simulink model "homework6"  (R2014b)
settings: Solver=ode45  StartTime=0.0  StopTime=10.0  RelTol=1e-3
values from neighbouring files (symbols this model uses):
  A = [-8.29e-2    0       -6.6e2   3.22e1 0, ... (first row only)    [hw6.m]
  B = [ 0      7.65, ... (first row only)    [hw6.m]
  C = [0     1 0 0 0, ... (first row only)    [hw6.m]
  D = [0 0, ... (first row only)    [hw6.m]
undefined symbols (not defined in the file or in its folder): sigbuilder_block
settings Model: Creator=karasinski  LastModifiedBy=karasinski

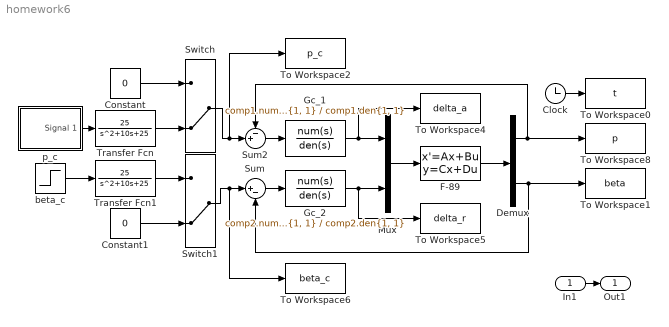
== system homework6 ==
  In1 : Inport
  Clock : Clock
  Constant : Constant  Value=0
  Constant1 : Constant  Value=0
  Demux : Demux  Outputs=2
  F-89 : StateSpace  A=A  B=B  C=C  D=D  X0=0
  Gc_1 : TransferFcn  Numerator=comp1.num{1, 1}  Denominator=comp1.den{1, 1}
  Gc_2 : TransferFcn  Numerator=comp2.num{1, 1}  Denominator=comp2.den{1, 1}
  Mux : Mux  Inputs=2
  Sum : Sum  Inputs=|+-
  Sum2 : Sum  Inputs=-+|
  Switch : ManualSwitch  CurrentSetting=0
  Switch1 : ManualSwitch  CurrentSetting=0
  To Workspace0 : ToWorkspace  VariableName=t  SampleTime=-1
  To Workspace1 : ToWorkspace  VariableName=beta  SampleTime=-1
  To Workspace2 : ToWorkspace  VariableName=p_c  SampleTime=-1
  To Workspace4 : ToWorkspace  VariableName=delta_a  SampleTime=-1
  To Workspace5 : ToWorkspace  VariableName=delta_r  SampleTime=-1
  To Workspace6 : ToWorkspace  VariableName=beta_c  SampleTime=-1
  To Workspace8 : ToWorkspace  VariableName=p  SampleTime=-1
  Transfer Fcn : TransferFcn  Numerator=[25]  Denominator=[1 10 25]
  Transfer Fcn1 : TransferFcn  Numerator=[25]  Denominator=[1 10 25]
  beta_c : Step  Time=0  After=5 / 57.3  SampleTime=0
  p_c : Subsystem  Tag=STV Subsys  LoadFcn=sigbuilder_block('load');  StartFcn=sigbuilder_block('start');  StopFcn=sigbuilder_block('stop');  ClipboardFcn=sigbuilder_block('clipboard');  mask(Sigbuilder block){}
      mask help: Simulink:masks:SigbuilderBlock_MD
      mask init:
      | if ~strcmp(get_param(bdroot(gcbh),'SimulationStatus'),'stopped') tuvar = sigbuilder_block('maskInit'); end
      settings: CopyFcn=sigbuilder_block('copy');  DeleteFcn=sigbuilder_block('delete');  ModelCloseFcn=sigbuilder_block('modelClose');  PreSaveFcn=sigbuilder_block('preSave');  PauseFcn=sigbuilder_block('pause');  ContinueFcn=sigbuilder_block('continue');  NameChangeFcn=sigbuilder_block('namechange');  OpenFcn=sigbuilder_block('open',[437.6 199.2 550.4 400 ]);  CloseFcn=sigbuilder_block('close');
      mask Display: plot(0, 0, 100, 100,[2, 2, 32, 32, 2], [68, 8, 8, 68, 68],[32, 2], [38, 38], [32, 19, 2],[53, 60, 44], [32, 17, 17, 2],[16, 16, 31, 31]);txt = getActiveGroup(gcbh);text(2, 100, txt,'verticalAlignment', 'top');
  Out1 : Outport
  wires:
  F-89/1 -> Demux/1
  Mux/1 -> F-89/1
  Clock/1 -> To Workspace0/1
  Gc_1/1 -> Mux/1, To Workspace4/1
  Gc_2/1 -> Mux/2, To Workspace5/1
  beta_c/1 -> Transfer Fcn1/1
  Sum/1 -> Gc_2/1
  Sum2/1 -> Gc_1/1
  Demux/1 -> Sum2/1, To Workspace8/1
  Demux/2 -> Sum/2, To Workspace1/1
  p_c/1(Signal 1) -> Transfer Fcn/1
  In1/1 -> Out1/1
  Switch/1 -> Sum2/2, To Workspace2/1
  Switch1/1 -> To Workspace6/1, Sum/1
  Constant/1 -> Switch/1
  Transfer Fcn1/1 -> Switch1/1
  Transfer Fcn/1 -> Switch/2
  Constant1/1 -> Switch1/2

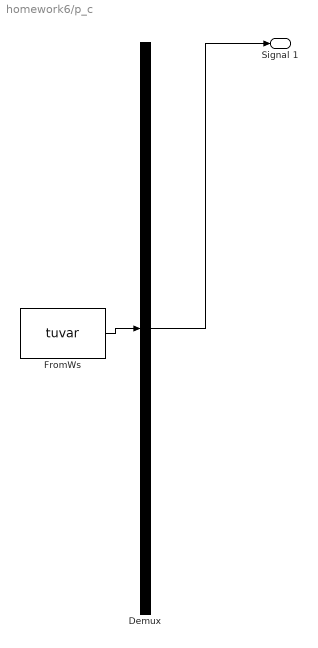
== system homework6/p_c ==
  Demux : Demux  Tag=STV Demux  Outputs=1
  FromWs : FromWorkspace  Tag=STV FromWs  VariableName=tuvar  SampleTime=0
      SigBuilderData=|
      | common.afterFinalStr = 'Extrapolate'
      | common.sampleTime = 0
      | dataSet.timeRange = [0 10]
      | dataSet.name = 'Group 1'
      | sbobj.Groups.Name = 'Group 1'
      | sbobj.Groups.Signals.Name = 'Signal 1'
      | sbobj.Groups.Signals.XData = [0 2 2 4 4 10]
      | sbobj.Groups.Signals.YData = [0.087260034904 0.087260034904 -0.087260034904 -0.087260034904 0 0]
  Signal 1 : Outport  Tag=STV Outport
  wires:
  Demux/1 -> Signal 1/1
  FromWs/1 -> Demux/1
